simulink model "chap4_2sim"  (Simulink 10.1)
settings: Solver=ode45  StartTime=0.0  StopTime=inf  FixedStep=0.001  RelTol=1e-3
settings Model: Creator=Administrator  LastModifiedBy=FIVE-CYCLE  ExtModeTrigMode=oneshot  ExtModeArmWhenConnect=off
settings DataIOCC: SignalLoggingName=sigsOut
settings OptimizationCC: BooleanDataType=off  OptimizeBlockIOStorage=off  BufferReuse=off  ExpressionFolding=off  ExpressionDepthLimit=2147483647  LocalBlockOutputs=off  InitFltsAndDblsToZero=on
settings DebuggingCC: SaveWithParameterizedLinksMsg=none  SignalResolutionControl=TryResolveAllWithWarning  MultiTaskDSMMsg=warning  MultiTaskCondExecSysMsg=none  FcnCallInpInsideContextMsg=warning  StateNameClashWarn=warning
settings HardwareCC: TargetUnknown=on
settings GRTTargetCC: TargetFcnLib=ansi_tfl_tmw.mat

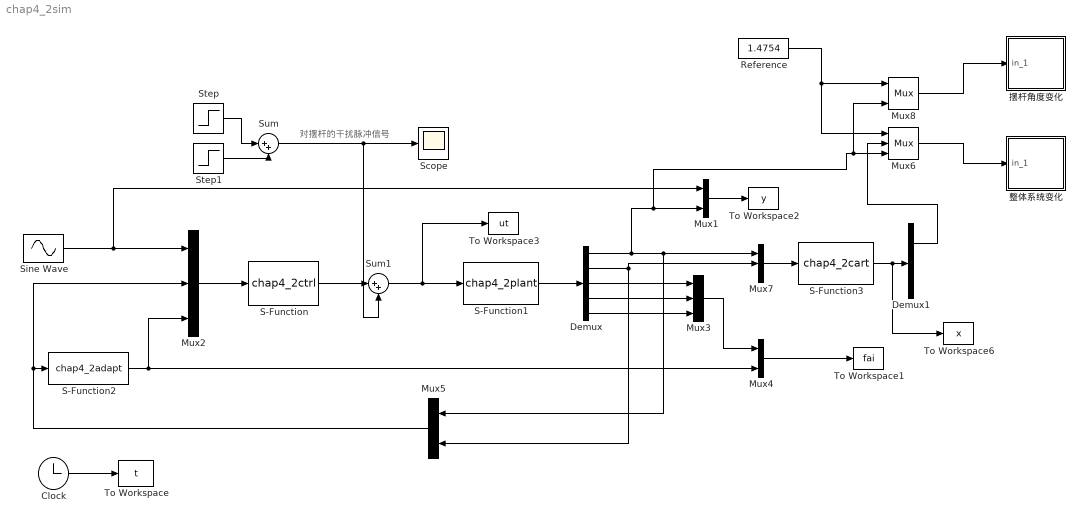
== system chap4_2sim ==
  note: 对摆杆的干扰脉冲信号
  Clock : Clock
  Demux : Demux  Outputs=5
      settings: DisplayOption=none
  Demux1 : Demux  Outputs=2
      settings: DisplayOption=none
  Mux1 : Mux  Inputs=2
  Mux{2..3,6..8} (5 alike) : Mux  Inputs=3
  Mux4 : Mux  Inputs=2
  Mux5 : Mux  Inputs=2
  Reference : Constant  Value=1.4754
  S-Function : S-Function  FunctionName=chap4_2ctrl  SFunctionDeploymentMode=off  EnableBusSupport=off
  S-Function1 : S-Function  FunctionName=chap4_2plant  SFunctionDeploymentMode=off  EnableBusSupport=off
  S-Function2 : S-Function  FunctionName=chap4_2adapt  SFunctionDeploymentMode=off  EnableBusSupport=off
  S-Function3 : S-Function  FunctionName=chap4_2cart  SFunctionDeploymentMode=off  EnableBusSupport=off
  Scope : Scope
  Sine Wave : Sin  Amplitude=0  Frequency=0.05  SampleTime=0
  Step : Step  Time=5  After=5  SampleTime=0
  Step1 : Step  Time=6  After=-5  SampleTime=0
  Sum : Sum  Inputs=|++
  Sum1 : Sum  Inputs=|++
  To Workspace : ToWorkspace  VariableName=t  SampleTime=-1
  To Workspace1 : ToWorkspace  VariableName=fai  SampleTime=-1
  To Workspace2 : ToWorkspace  VariableName=y  SampleTime=-1
  To Workspace3 : ToWorkspace  VariableName=ut  SampleTime=-1
  To Workspace6 : ToWorkspace  VariableName=x  SampleTime=-1
  摆杆角度变化 : Subsystem  mask(Pendulum plot){RefBlock=Reference}
      mask prompts: RefBlock "DC reference signal block name:"
      mask help: Pendulum plot
      mask Help: Pendulum animation function using Handle graphics.
      mask Display: plot([-10 10],[0 0],[-2 -2 2 2],[0 1 1 0],[0 3],[1 5])
  整体系统变化 : Subsystem  mask(Pendulum plot){RefBlock=Reference}
      mask prompts: RefBlock "DC reference signal block name:"
      mask help: Pendulum plot
      mask Help: Pendulum animation function using Handle graphics.
      mask Display: plot([-10 10],[0 0],[-2 -2 2 2],[0 1 1 0],[0 3],[1 5])
  wires:
  Clock/1 -> To Workspace/1
  Sine Wave/1 -> Mux1/1, Mux2/1
  Mux1/1 -> To Workspace2/1
  Mux2/1 -> S-Function/1
  S-Function1/1 -> Demux/1
  Demux/1 -> Mux8/3, Mux6/3, Mux1/2, Mux7/1, Mux5/1
  Demux/3 -> Mux3/1
  Demux/4 -> Mux3/2
  Demux/5 -> Mux3/3
  Mux4/1 -> To Workspace1/1
  Mux3/1 -> Mux4/1
  Demux/2 -> Mux7/2, Mux5/2
  Mux5/1 -> Mux2/2, S-Function2/1
  S-Function2/1 -> Mux2/3, Mux4/2
  Mux6/1 -> 整体系统变化/1(in_1)
  Mux7/1 -> S-Function3/1
  Reference/1 -> Mux6/1, Mux8/1
  S-Function3/1 -> To Workspace6/1, Demux1/1
  Demux1/1 -> Mux6/2
  Mux8/1 -> 摆杆角度变化/1(in_1)
  Step1/1 -> Sum/2
  Step/1 -> Sum/1
  Sum/1 -> Sum1/2, Scope/1
  S-Function/1 -> Sum1/1
  Sum1/1 -> To Workspace3/1, S-Function1/1

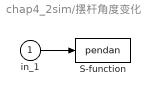
== system chap4_2sim/摆杆角度变化 ==
  in_1 : Inport
  S-function : S-Function  FunctionName=pendan  Parameters=RefBlock  SFunctionDeploymentMode=off  EnableBusSupport=off
      settings: DeleteFcn=pendan([],[],[],'DeleteBlock');
  wires:
  in_1/1 -> S-function/1

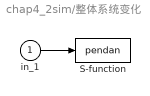
== system chap4_2sim/整体系统变化 ==
  in_1 : Inport
  S-function : S-Function  FunctionName=pendan  Parameters=RefBlock  SFunctionDeploymentMode=off  EnableBusSupport=off
      settings: DeleteFcn=pendan([],[],[],'DeleteBlock');
  wires:
  in_1/1 -> S-function/1
